simulink model "Model"  (R2018a)
settings: Solver=ode5  StartTime=0.0  StopTime=1000  FixedStep=0.05  RelTol=1e-3
settings Model: PacingRate=100  Creator=Hungs  LastModifiedBy=Hungs

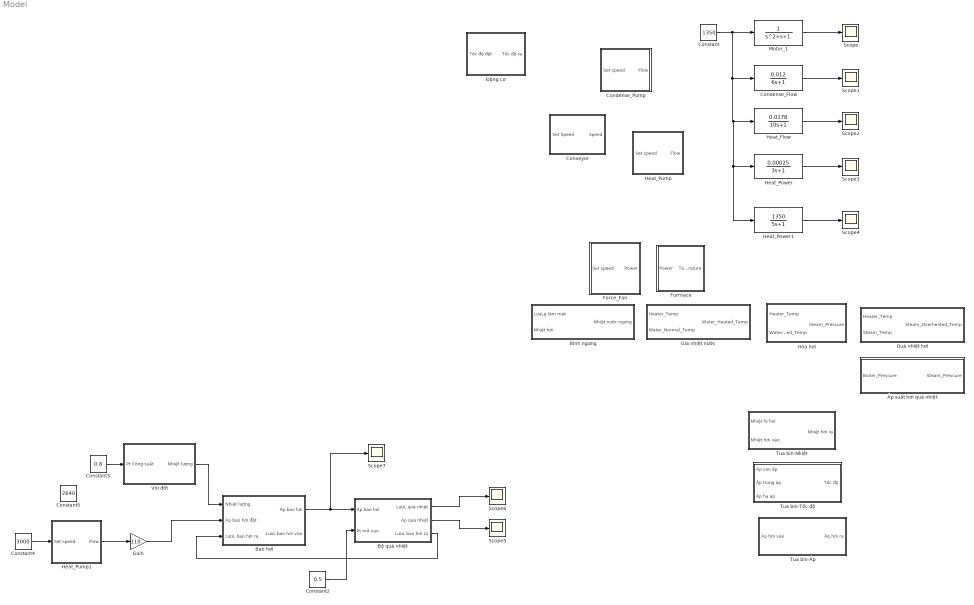
== system Model ==
  Bao hơi : Subsystem  mask{Cm=0.3, Kw=0.04, Kt=0.000025, Kh=-300, Cd=150}
      mask prompts: Cm "Hệ số hấp thụ nhiệt ống sinh hơi"; Kw "Hệ số truyền nhiệt ống sinh hơi"; Kt "Tỉ lệ áp suất - nhiệt độ trong ống sinh hơi"; Kh "Hệ số biến thiên entanpi theo áp suất bao hơi"; Cd "Thời hằng bao hơi"
  Bình ngưng : Subsystem
  Bộ quá nhiệt : Subsystem  mask{K=44, Cs=20}
      mask prompts: K "Hệ số tụt áp"; Cs "Thời hằng bộ quá nhiệt"
  Condense_Flow : TransferFcn  Numerator=[0.012]  Denominator=[6 1]
  Condense_Pump : Subsystem
      mask Display: image('C:\Program Files\MATLAB\ThermalElectricity\Maskicon\Pump.png');
  Constant : Constant  Value=1350
  Constant2 : Constant  Value=0.5
  Constant3 : Constant  Value=0.8
  Constant4 : Constant  Value=3000
  Constant5 : Constant  Value=2640
  Conveyor : Subsystem
      mask Display: image('C:\Program Files\MATLAB\ThermalElectricity\Maskicon\conveyor.png');
  Force_Fan : Subsystem
      mask Display: image('C:\Program Files\MATLAB\ThermalElectricity\Maskicon\Fan.png');
  Furrnace : Subsystem
      mask Display: image('C:\Program Files\MATLAB\ThermalElectricity\Maskicon\Furnace.png');
  Gain : Gain  Gain=110
  Gia nhiệt nước : Subsystem
  Heat_Flow : TransferFcn  Numerator=[0.0178]  Denominator=[10 1]
  Heat_Power : TransferFcn  Numerator=[0.00025]  Denominator=[3 1]
  Heat_Power1 : TransferFcn  Numerator=[1350]  Denominator=[5 1]
  Heat_Pump : Subsystem
      mask Display: image('C:\Program Files\MATLAB\ThermalElectricity\Maskicon\Pump.png');
  Heat_Pump1 : Subsystem
      mask Display: image('C:\Program Files\MATLAB\ThermalElectricity\Maskicon\Pump.png');
  Hóa hơi : Subsystem
  Motor_1 : TransferFcn  Denominator=[1 1 1]
  Quá nhiệt hơi : Subsystem
  Scope{,1..7} (8 alike) : Scope
  Tua bin-Nhiệt : Subsystem
  Tua bin-Tốc độ : Subsystem
  Tua bin-Áp : Subsystem
  Vòi đốt : Subsystem  mask{Tf=100, Td=20}
      mask prompts: Tf "Thời hằng vòi đốt"; Td "Thời gian trễ vòi đốt"
  Áp suất hơi quá nhiệt : Subsystem
  Động cơ : Subsystem
  wires:
  Motor_1/1 -> Scope/1
  Condense_Flow/1 -> Scope1/1
  Heat_Flow/1 -> Scope2/1
  Constant/1 -> Heat_Power1/1, Heat_Power/1, Heat_Flow/1, Condense_Flow/1, Motor_1/1
  Heat_Power/1 -> Scope3/1
  Heat_Power1/1 -> Scope4/1
  Vòi đốt/1(Nhiệt lượng) -> Bao hơi/1(Nhiệt lượng)
  Bao hơi/1(Áp bao hơi) -> Bộ quá nhiệt/1(Áp bao hơi), Scope7/1
  Bộ quá nhiệt/3(LưuL bao hơi ra) -> Bao hơi/3(LưuL bao hơi ra)
  Gain/1 -> Bao hơi/2(Áp bao hơi đặt)
  Constant2/1 -> Bộ quá nhiệt/2(Pt mở van)
  Bộ quá nhiệt/2(Áp quá nhiệt) -> Scope5/1
  Constant3/1 -> Vòi đốt/1(Pt Công suất)
  Bộ quá nhiệt/1(LưuL quá nhiệt) -> Scope6/1
  Constant4/1 -> Heat_Pump1/1(Set speed)
  Heat_Pump1/1(Flow) -> Gain/1

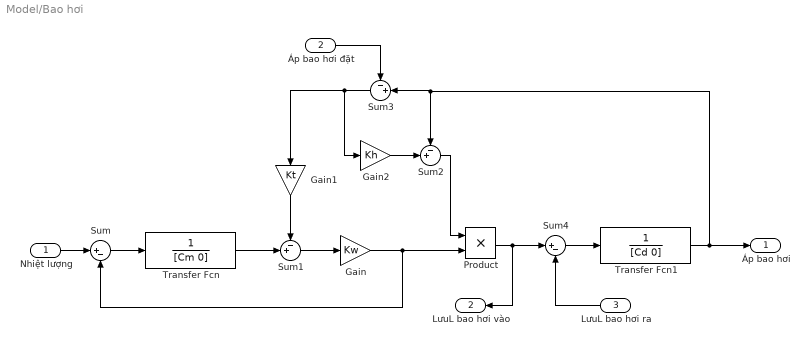
== system Model/Bao hơi ==
  Nhiệt lượng : Inport
  Áp bao hơi đặt : Inport  Port=2
  LưuL bao hơi ra : Inport  Port=3
  Gain : Gain  Gain=Kw
  Gain1 : Gain  Gain=Kt
  Gain2 : Gain  Gain=Kh
  Product : Product
  Sum : Sum  Inputs=|+-
  Sum1 : Sum  Inputs=-+|
  Sum2 : Sum  Inputs=-+|
  Sum3 : Sum  Inputs=-+|
  Sum4 : Sum  Inputs=|+-
  Transfer Fcn : TransferFcn  Denominator=[Cm 0]
  Transfer Fcn1 : TransferFcn  Denominator=[Cd 0]
  Áp bao hơi : Outport
  LưuL bao hơi vào : Outport  Port=2
  wires:
  Transfer Fcn/1 -> Sum1/2
  Sum1/1 -> Gain/1
  Gain/1 -> Product/2, Sum/2
  Sum/1 -> Transfer Fcn/1
  Gain1/1 -> Sum1/1
  Nhiệt lượng/1 -> Sum/1
  Transfer Fcn1/1 -> Áp bao hơi/1, Sum2/1, Sum3/2
  Sum2/1 -> Product/1
  Gain2/1 -> Sum2/2
  Sum3/1 -> Gain1/1, Gain2/1
  Áp bao hơi đặt/1 -> Sum3/1
  Product/1 -> Sum4/1, LưuL bao hơi vào/1
  LưuL bao hơi ra/1 -> Sum4/2
  Sum4/1 -> Transfer Fcn1/1

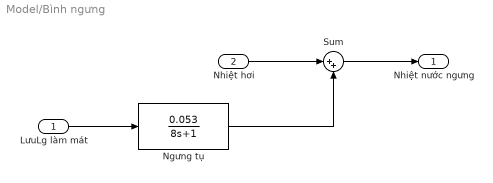
== system Model/Bình ngưng ==
  LưuLg làm mát : Inport
  Nhiệt hơi : Inport  Port=2
  Ngưng tụ : TransferFcn  Numerator=[0.053]  Denominator=[8 1]
  Sum : Sum  Inputs=|++
  Nhiệt nước ngưng : Outport
  wires:
  Sum/1 -> Nhiệt nước ngưng/1
  Ngưng tụ/1 -> Sum/2
  Nhiệt hơi/1 -> Sum/1
  LưuLg làm mát/1 -> Ngưng tụ/1

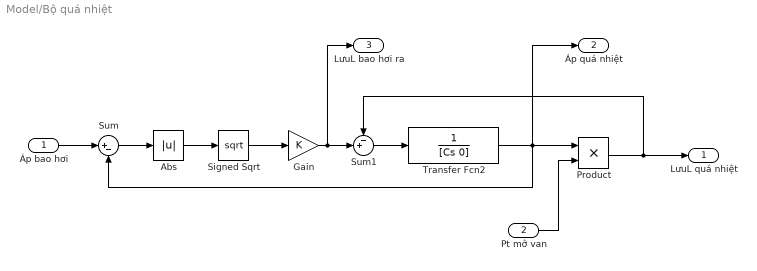
== system Model/Bộ quá nhiệt ==
  Áp bao hơi : Inport
  Pt mở van : Inport  Port=2
  Abs : Abs
  Gain : Gain  Gain=K
  Product : Product
  Signed Sqrt : Sqrt  SaturateOnIntegerOverflow=on
  Sum : Sum  Inputs=|+-
  Sum1 : Sum  Inputs=-+|
  Transfer Fcn2 : TransferFcn  Denominator=[Cs 0]
  LưuL quá nhiệt : Outport
  Áp quá nhiệt : Outport  Port=2
  LưuL bao hơi ra : Outport  Port=3
  wires:
  Transfer Fcn2/1 -> Áp quá nhiệt/1, Sum/2, Product/1
  Áp bao hơi/1 -> Sum/1
  Sum/1 -> Abs/1
  Abs/1 -> Signed Sqrt/1
  Signed Sqrt/1 -> Gain/1
  Pt mở van/1 -> Product/2
  Gain/1 -> LưuL bao hơi ra/1, Sum1/2
  Sum1/1 -> Transfer Fcn2/1
  Product/1 -> LưuL quá nhiệt/1, Sum1/1

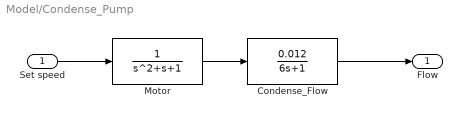
== system Model/Condense_Pump ==
  Set speed : Inport
  Condense_Flow : TransferFcn  Numerator=[0.012]  Denominator=[6 1]
  Motor : TransferFcn  Denominator=[1 1 1]
  Flow : Outport
  wires:
  Motor/1 -> Condense_Flow/1
  Set speed/1 -> Motor/1
  Condense_Flow/1 -> Flow/1

== system Model/Conveyor ==
  Set Speed : Inport
  Motor_1 : TransferFcn  Denominator=[1 1 1]
  Speed : Outport
  wires:
  Set Speed/1 -> Motor_1/1
  Motor_1/1 -> Speed/1

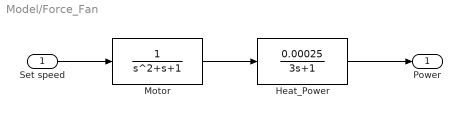
== system Model/Force_Fan ==
  Set speed : Inport
  Heat_Power : TransferFcn  Numerator=[0.00025]  Denominator=[3 1]
  Motor : TransferFcn  Denominator=[1 1 1]
  Power : Outport
  wires:
  Motor/1 -> Heat_Power/1
  Set speed/1 -> Motor/1
  Heat_Power/1 -> Power/1

== system Model/Furrnace ==
  Power : Inport
  Furnace : TransferFcn  Numerator=[1350]  Denominator=[5 1]
  Temperature : Outport
  wires:
  Furnace/1 -> Temperature/1
  Power/1 -> Furnace/1

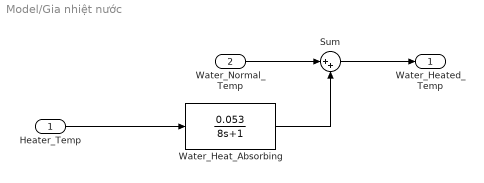
== system Model/Gia nhiệt nước ==
  Heater_Temp : Inport
  Water_Normal_Temp : Inport  Port=2
  Sum : Sum  Inputs=|++
  Water_Heat_Absorbing : TransferFcn  Numerator=[0.053]  Denominator=[8 1]
  Water_Heated_Temp : Outport
  wires:
  Heater_Temp/1 -> Water_Heat_Absorbing/1
  Water_Normal_Temp/1 -> Sum/1
  Water_Heat_Absorbing/1 -> Sum/2
  Sum/1 -> Water_Heated_Temp/1

== system Model/Heat_Pump ==
  Set speed : Inport
  Heat_Flow : TransferFcn  Numerator=[0.0178]  Denominator=[10 1]
  Motor : TransferFcn  Denominator=[1 1 1]
  Flow : Outport
  wires:
  Heat_Flow/1 -> Flow/1
  Set speed/1 -> Motor/1
  Motor/1 -> Heat_Flow/1

== system Model/Heat_Pump1 ==
  Set speed : Inport
  Heat_Flow : TransferFcn  Numerator=[0.0178]  Denominator=[10 1]
  Motor : TransferFcn  Denominator=[1 1 1]
  Flow : Outport
  wires:
  Heat_Flow/1 -> Flow/1
  Set speed/1 -> Motor/1
  Motor/1 -> Heat_Flow/1

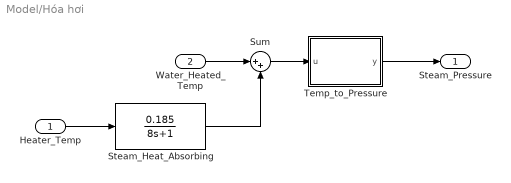
== system Model/Hóa hơi ==
  Heater_Temp : Inport
  Water_Heated_Temp : Inport  Port=2
  Steam_Heat_Absorbing : TransferFcn  Numerator=[0.185]  Denominator=[8 1]
  Sum : Sum  Inputs=|++
  Temp_to_Pressure : MATLAB Function  TreatAsAtomicUnit=on
  Steam_Pressure : Outport
  wires:
  Sum/1 -> Temp_to_Pressure/1(u)
  Steam_Heat_Absorbing/1 -> Sum/2
  Water_Heated_Temp/1 -> Sum/1
  Heater_Temp/1 -> Steam_Heat_Absorbing/1
  Temp_to_Pressure/1(y) -> Steam_Pressure/1

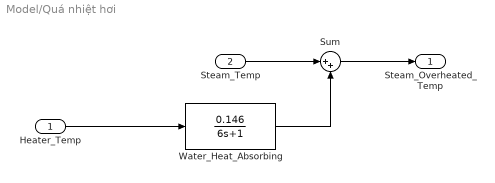
== system Model/Quá nhiệt hơi ==
  Heater_Temp : Inport
  Steam_Temp : Inport  Port=2
  Sum : Sum  Inputs=|++
  Water_Heat_Absorbing : TransferFcn  Numerator=[0.146]  Denominator=[6 1]
  Steam_Overheated_Temp : Outport
  wires:
  Sum/1 -> Steam_Overheated_Temp/1
  Water_Heat_Absorbing/1 -> Sum/2
  Steam_Temp/1 -> Sum/1
  Heater_Temp/1 -> Water_Heat_Absorbing/1

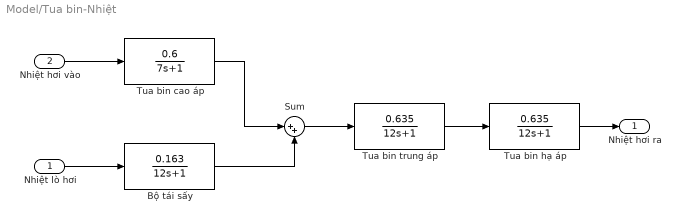
== system Model/Tua bin-Nhiệt ==
  Nhiệt lò hơi : Inport
  Nhiệt hơi vào : Inport  Port=2
  Bộ tái sấy : TransferFcn  Numerator=[0.163]  Denominator=[12 1]
  Sum : Sum  Inputs=|++
  Tua bin cao áp : TransferFcn  Numerator=[0.6]  Denominator=[7 1]
  Tua bin hạ áp : TransferFcn  Numerator=[0.635]  Denominator=[12 1]
  Tua bin trung áp : TransferFcn  Numerator=[0.635]  Denominator=[12 1]
  Nhiệt hơi ra : Outport
  wires:
  Nhiệt lò hơi/1 -> Bộ tái sấy/1
  Bộ tái sấy/1 -> Sum/2
  Nhiệt hơi vào/1 -> Tua bin cao áp/1
  Tua bin cao áp/1 -> Sum/1
  Sum/1 -> Tua bin trung áp/1
  Tua bin trung áp/1 -> Tua bin hạ áp/1
  Tua bin hạ áp/1 -> Nhiệt hơi ra/1

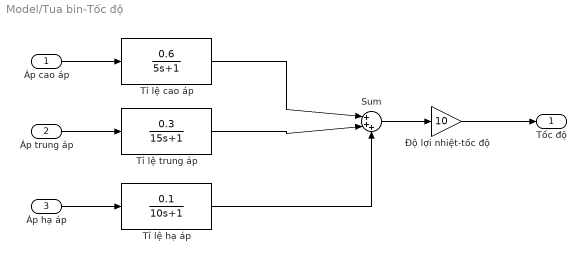
== system Model/Tua bin-Tốc độ ==
  Áp cao áp : Inport
  Áp trung áp : Inport  Port=2
  Áp hạ áp : Inport  Port=3
  Sum : Sum  Inputs=|+++
  Tỉ lệ cao áp : TransferFcn  Numerator=[0.6]  Denominator=[5 1]
  Tỉ lệ hạ áp : TransferFcn  Numerator=[0.1]  Denominator=[10 1]
  Tỉ lệ trung áp : TransferFcn  Numerator=[0.3]  Denominator=[15 1]
  Độ lợi nhiệt-tốc độ : Gain  Gain=10
  Tốc độ : Outport
  wires:
  Áp cao áp/1 -> Tỉ lệ cao áp/1
  Tỉ lệ cao áp/1 -> Sum/1
  Sum/1 -> Độ lợi nhiệt-tốc độ/1
  Áp trung áp/1 -> Tỉ lệ trung áp/1
  Áp hạ áp/1 -> Tỉ lệ hạ áp/1
  Tỉ lệ trung áp/1 -> Sum/2
  Tỉ lệ hạ áp/1 -> Sum/3
  Độ lợi nhiệt-tốc độ/1 -> Tốc độ/1

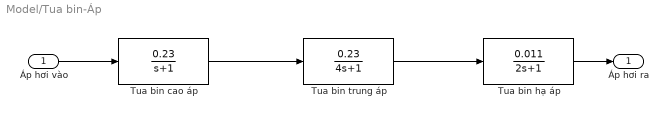
== system Model/Tua bin-Áp ==
  Áp hơi vào : Inport
  Tua bin cao áp : TransferFcn  Numerator=[0.23]  Denominator=[1 1]
  Tua bin hạ áp : TransferFcn  Numerator=[0.011]  Denominator=[2 1]
  Tua bin trung áp : TransferFcn  Numerator=[0.23]  Denominator=[4 1]
  Áp hơi ra : Outport
  wires:
  Tua bin hạ áp/1 -> Áp hơi ra/1
  Tua bin trung áp/1 -> Tua bin hạ áp/1
  Tua bin cao áp/1 -> Tua bin trung áp/1
  Áp hơi vào/1 -> Tua bin cao áp/1

== system Model/Vòi đốt ==
  Pt Công suất : Inport
  Furnace : TransferFcn  Denominator=[Tf 1]
  Transport Delay : TransportDelay  DelayTime=Td
  Nhiệt lượng : Outport
  wires:
  Pt Công suất/1 -> Furnace/1
  Furnace/1 -> Transport Delay/1
  Transport Delay/1 -> Nhiệt lượng/1

== system Model/Áp suất hơi quá nhiệt ==
  Boiler_Pressure : Inport
  Overheated_Pressure : TransferFcn  Numerator=[1.1]  Denominator=[2 1]
  Steam_Pressure : Outport
  wires:
  Boiler_Pressure/1 -> Overheated_Pressure/1
  Overheated_Pressure/1 -> Steam_Pressure/1

== system Model/Động cơ ==
  Tốc độ đặt : Inport
  Bão hòa 2 cực : Saturate  UpperLimit=1500  LowerLimit=0
  Động cơ AC : TransferFcn  Denominator=[1 1 1]
  Tốc độ ra : Outport
  wires:
  Bão hòa 2 cực/1 -> Tốc độ ra/1
  Tốc độ đặt/1 -> Động cơ AC/1
  Động cơ AC/1 -> Bão hòa 2 cực/1

== matlab function Model/Hóa hơi/Temp_to_Pressure ==
  data: u input; y output
function y = fcn(u)
to = [29.95 32.89 41.53 45.82 52.57 60.08 69.12 75.87 81.33 93.5 99.62 109.32 ...
    120.24 133.56 143.64 151.87 158.86 164.98 170.44 175.39 179.92 195.08 212.42 ...
    233.89 250.39 263.98 285.86 311.03 342.34 357.04 365.80 373.70];
p = [0.004 0.005 0.008 0.01 0.018 0.02 0.03 0.04 0.05 0.08 0.1 0.14 0.2 0.3 0.4 ...
    0.5 0.6 0.7 0.8 0.9 1 1.4 2 3 4 5 7 10 15 18 20 22];
y = interp1(to,p,u);
